simulink model "preview_control"  (R2014b)
settings: Solver=FixedStepDiscrete  StartTime=0.0  StopTime=sim_time  FixedStep=T  MaxStep=1e-4  RelTol=1e-6
values from neighbouring files (symbols this model uses):
  desired_zmp = [t' desired_zmp']    [cart_table.m]    (also in preview_control_c.m)
  g = 9.8    [cart_table.m]    (also in preview_control_c.m; preview_control_params.m)
  Kx = KK(1,2:4)    [preview_control_params.m]
  N = 16000    [cart_table.m]    (also in preview_control_c.m)
  T = 1e-4    (= 0.0001)    [cart_table.m]    (also in preview_control_c.m)
  Zc = 1    [cart_table.m]    (also in preview_control_c.m)
libraries: simulink x2
settings Model: Creator=StipudUser  LastModifiedBy=aelphy
settings SolverCC: AlgebraicLoopSolver=LineSearch

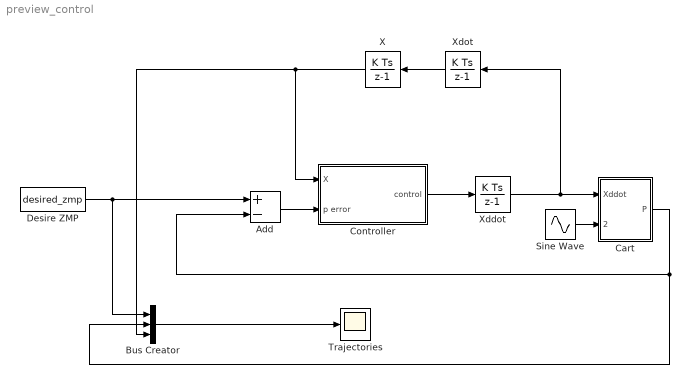
== system preview_control ==
  Add : Sum  Inputs=+-
  Bus Creator : BusCreator  Inputs=3
  Cart : Subsystem
  "Controller " : Subsystem
  "Desire ZMP " : FromWorkspace  VariableName=desired_zmp  SampleTime=T  OutputAfterFinalValue=Setting to zero
  Sine Wave : Sin  Amplitude=0  Bias=Zc  Frequency=2  SampleTime=T
  Trajectories : Scope
      settings: TickLabels=on  ShowLegends=on  TimeRange=0.01075847229693316  YMin=-0.00012  YMax=0  MaxDataPoints=500000  SampleInput=on
  X : DiscreteIntegrator  SampleTime=-1
  Xddot : DiscreteIntegrator  SampleTime=-1
  Xdot : DiscreteIntegrator  SampleTime=-1
  wires:
  Cart/1("P ") -> Bus Creator/2, Add/2
  "Controller "/1(control) -> Xddot/1
  Add/1 -> "Controller "/2(p error)
  "Desire ZMP "/1 -> Add/1, Bus Creator/1
  Sine Wave/1 -> Cart/2("Y_CoM ")
  Xddot/1 -> Cart/1("Xddot "), Xdot/1
  Xdot/1 -> X/1
  X/1 -> Bus Creator/3, "Controller "/1(X)
  Bus Creator/1 -> Trajectories/1

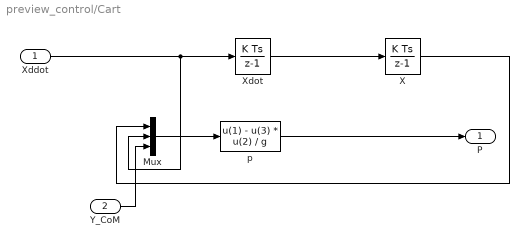
== system preview_control/Cart ==
  "Xddot " : Inport
  "Y_CoM " : Inport  Port=2
  Mux : Mux  Inputs=3
  X : DiscreteIntegrator  SampleTime=-1
  "Xdot " : DiscreteIntegrator  SampleTime=-1
  p : Fcn  Expr=u(1) - u(3) * u(2) / g
  "P " : Outport
  wires:
  p/1 -> "P "/1
  Mux/1 -> p/1
  "Xdot "/1 -> X/1
  X/1 -> Mux/1
  "Y_CoM "/1 -> Mux/3
  "Xddot "/1 -> "Xdot "/1, Mux/2

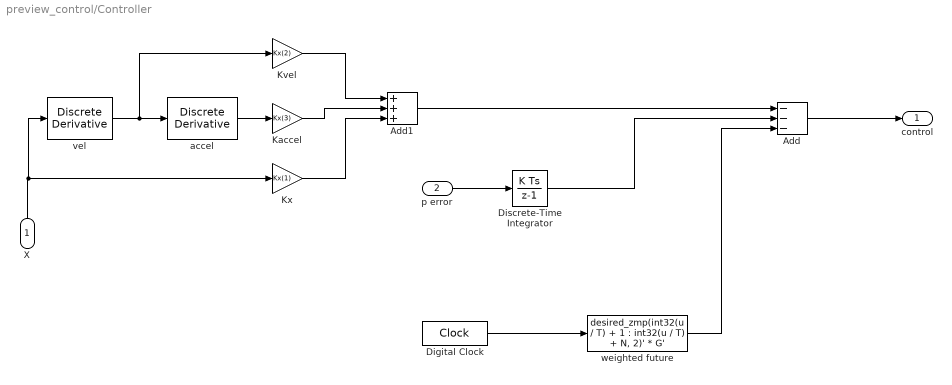
== system preview_control/Controller  ==
  X : Inport
  p error : Inport  Port=2
  Add : Sum  Inputs=---
  Add1 : Sum  Inputs=+++
  Digital Clock : DigitalClock  SampleTime=T
  Discrete-Time Integrator : DiscreteIntegrator  gainval=Ke  InitialConditionSetting=State (most efficient)  SampleTime=T
  Kaccel : Gain  Gain=Kx(3)  SampleTime=T
  Kvel : Gain  Gain=Kx(2)  SampleTime=T
  Kx : Gain  Gain=Kx(1)  SampleTime=T
  accel : simulink/Discrete/Discrete Derivative  gainval=1.0  ICPrevScaledInput=0.0  InputProcessing=Inherited  OutMin=[]  OutMax=[]  OutDataType=fixdt(1, 16)  OutScaling=2^-10  DoSatur=off
  vel : simulink/Discrete/Discrete Derivative  gainval=1.0  ICPrevScaledInput=0.0  InputProcessing=Inherited  OutMin=[]  OutMax=[]  OutDataType=fixdt(1, 16)  OutScaling=2^-10  DoSatur=off
  weighted future : MATLABFcn  MATLABFcn=desired_zmp(int32(u / T) + 1 : int32(u / T) + N, 2)' * G'  SampleTime=T
  control : Outport
  wires:
  Add/1 -> control/1
  p error/1 -> Discrete-Time Integrator/1
  Discrete-Time Integrator/1 -> Add/2
  X/1 -> Kx/1, vel/1
  vel/1 -> Kvel/1, accel/1
  accel/1 -> Kaccel/1
  Kx/1 -> Add1/3
  Kaccel/1 -> Add1/2
  Kvel/1 -> Add1/1
  Add1/1 -> Add/1
  weighted future/1 -> Add/3
  Digital Clock/1 -> weighted future/1
